simulink library "NSA_DEVS_LOGISTICS"  (R2025a)
settings: Solver=VariableStepAuto  StartTime=0.0  StopTime=10.0  RelTol=1e-3
libraries: $bdroot x9, NSA_DEVS_MATH_OPERATIONS x3, NSA_DEVS_ROUTING x1
settings Model: Creator=david  LastModifiedBy=peter
settings OptimizationCC: ReuseModelBlockBuffer=off
settings RTWCC: GPUComputeCapability=3.5

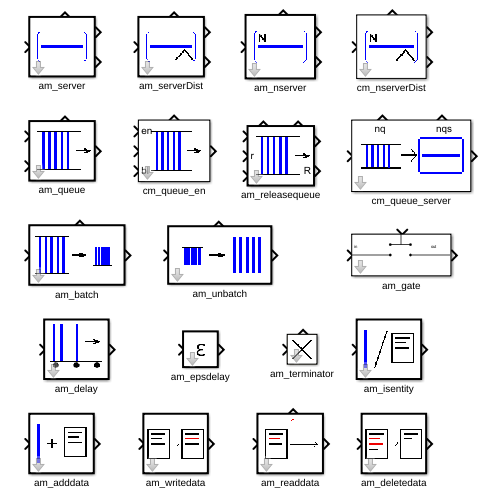
[thumbnail: Simulink's stored preview of the top-level diagram]
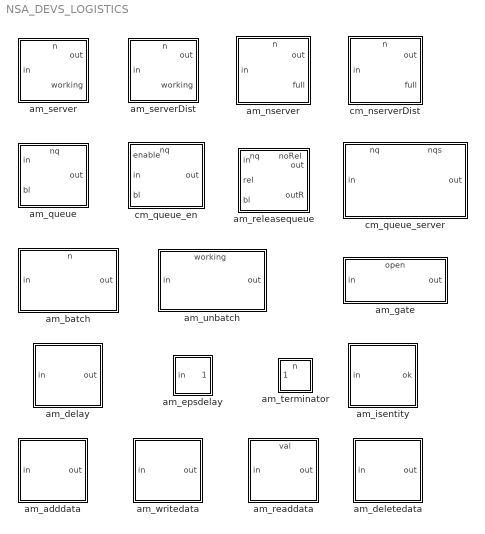
== system NSA_DEVS_LOGISTICS ==
  am_adddata : Subsystem  TreatAsAtomicUnit=on  mask(Adddata){fields=["name", "age"], values=["Peter", 42], numeric=[false, true], infield="id", tau=[0,1], debug=0}
      mask prompts: fields "field names"; values "field values"; numeric "flags to denote numeric values"; infield "field name of input value"
      mask help: Adds data fields to the input object.
      mask Help:
      | <p>Adds data fields to the input object.<br>
      | If the input is a struct, the new fields are added to the struct.
      | Otherwise a new struct is created and the incoming value is stored in an extra field.</p>
      | 
      | <p>Ports
      | <ul>
      | <li>inputs:
      |   <ul>
      |     <li>in: incoming value</li>
      |   </ul>
      | </li>
      | <li>outputs:
      |   <ul>
      |     <li>out: outgoing entity</li>
      |   </ul>
      | </li>
      | </ul>
      | </p>
      | 
      | <p>System Parameters
      | <ul>
      | <li>fields:  vector of new field names</li>
      | <li>values:  vector of corresponding values</li>
      | <li>numeric:  vector of booleans denoting numerical fields</li>
      | <li>infield:  field name for incoming value (if not a struct)</li>
      | <li>tau:   infinitesimal delay</li>
      | <li>debug: flag to enable debug information</li>
      | </ul>
      | </p>
      | 
      | <p>States
      | <ul>
      | <li>s:   running</li>
      | </ul>
      | </p>
      mask DialogControl Container4 Prompt: General
      mask DialogControl Container5 Prompt: Advanced
      mask Display: image('icon_adddata.png');
  am_batch : Subsystem  TreatAsAtomicUnit=on  mask(Batch){N=10, tau=[0,1], debug=0}
      mask prompts: N "batch size"
      mask help: Combine N entities to one batch entity.
      settings: PortSchema="{\"entries\":[{\"content\":{\"sides\":[{\"content\":{\"connectorIds\":[\"In1\"]},\"type\":\"ConnectorPlacement.EquallySpacedRectSide\",\"uuid\":\"8e15954b-329c-42af-8049-37e3c5654def\"},{\"content\":{\"connectorIds\":[\"Out1\"],\"side\":\"RIGHT\"},\"type\":\"ConnectorPlacement.EquallySpacedRectSide\",\"uuid\":\"63417118-70ef-43c0-aba5-016625c71a51\"},{\"content\":{\"connectorIds\":[\"Out2\"],\"side\":\"TOP\"},\"type\":\"ConnectorPlacement.EquallySpacedRectSide\",\"uuid\":\"b4e4d2cb-0431-4da8-a13e-061eb074f0ba\"}]},\"type\":\"ConnectorPlacement.EquallySpacedConnector\",\"uuid\":\"10cbbf1b-ecfb-492d-a1e3-9fcc3fe586bb\"}],\"packageUris\":[\"http://schema.mathworks.com/mf0/Connector/R2020b\"],\"version\":\"1.0\"}"
      mask Help:
      | <p>Combine N entities to one batch entity.</p>
      | 
      | <p>Ports
      | <ul>
      | <li>inputs:
      |   <ul>
      |     <li>in: incoming entities</li>
      |   </ul>
      | </li>
      | <li>outputs:
      |   <ul>
      |     <li>out: outgoing entities</li>
      |     <li>n: current internal batch size</li>
      |   </ul>
      | </li>
      | </ul>
      | </p>
      | 
      | <p>System Parameters
      | <ul>
      | <li>N:  number of input entities to be combined to one output batch</li>
      | <li>tau:   infinitesimal delay</li>
      | <li>debug: flag to enable debug information</li>
      | </ul>
      | </p>
      | 
      | <p>States
      | <ul>
      | <li>s:   running</li>
      | <li>E:  collection of incoming entities</li>
      | <li>n:  current number of internal entities</li>
      | </ul>
      | </p>
      mask DialogControl Container3 Prompt: General
      mask DialogControl Container4 Prompt: Advanced
      mask Display: image('icon_batch.png');
  am_delay : Subsystem  TreatAsAtomicUnit=on  mask(Delay){dt=[1,0], tau=[0,1], debug=0}
      mask prompts: dt "delay time"
      mask help: Delays the input signal by a constant amount.
      mask Help:
      | <p>Delays the input entities by a constant amount.</p>
      | 
      | <p>Ports
      | <ul>
      | <li>inputs:
      |   <ul>
      |     <li>in: incoming entities</li>
      |   </ul>
      | </li>
      | <li>outputs:
      |   <ul>
      |     <li>out: outgoing entities</li>
      |   </ul>
      | </li>
      | </ul>
      | </p>
      | 
      | <p>System Parameters
      | <ul>
      | <li>dt:  delay time</li>
      | <li>tau:   infinitesimal delay</li>
      | <li>debug: flag to enable debug information</li>
      | </ul>
      | </p>
      | 
      | <p>States
      | <ul>
      | <li>s:   running</li>
      | <li>E:  waiting input values, <br>E(i).x = value, E(i).e = remaining waiting time</li>
      | </ul>
      | </p>
      mask DialogControl Container4 Prompt: General
      mask DialogControl Container5 Prompt: Advanced
      mask Display: image('icon_delay.png');
  am_deletedata : Subsystem  TreatAsAtomicUnit=on  mask(Deletedata){fields="tS", tau=[0,1], debug=0}
      mask prompts: fields "fields to delete"
      mask help: Deletes data fields from the input object.
      mask Help:
      | <p>Deletes data fields from the input object.</p>
      | 
      | <p>Ports
      | <ul>
      | <li>inputs:
      |   <ul>
      |     <li>in: incoming entity</li>
      |   </ul>
      | </li>
      | <li>outputs:
      |   <ul>
      |     <li>out: outgoing entity</li>
      |   </ul>
      | </li>
      | </ul>
      | </p>
      | 
      | <p>System Parameters
      | <ul>
      | <li>fields:   vector of field names to be deleted</li>
      | <li>tau:   infinitesimal delay</li>
      | <li>debug: flag to enable debug information</li>
      | </ul>
      | </p>
      | 
      | <p>States
      | <ul>
      | <li>s:   running</li>
      | </ul>
      | </p>
      mask DialogControl Container4 Prompt: General
      mask DialogControl Container5 Prompt: Advanced
      mask Display: image('icon_deletedata.png');
  am_epsdelay : Subsystem  TreatAsAtomicUnit=on  mask(EpsDelay){tau=[0,1], debug=0}
      mask help: Delays its input by an infinitesimal amount.
      mask Help:
      | <p>Delays its input by an infinitesimal amount.</p>
      | 
      | <p>Ports
      | <ul>
      | <li>inputs:
      |   <ul>
      |     <li>in: incoming value or entity</li>
      |   </ul>
      | </li>
      | <li>outputs:
      |   <ul>
      |     <li>out: outgoing value or entity</li>
      |   </ul>
      | </li>
      | </ul>
      | </p>
      | 
      | <p>System Parameters
      | <ul>
      | <li>debug: flag to enable debug information</li>
      | <li>tau:   infinitesimal delay</li>
      | </ul>
      | </p>
      | 
      | <p>States
      | <ul>
      | <li>s:   running</li>
      | </ul>
      | </p>
      mask DialogControl Container5 Prompt: Advanced
      mask Display: image('icon_epsdelay.png');
  am_gate : Subsystem  mask(Gate){isOpen0=false, tau_copy_copy=[0,1], debug_copy_copy=0}
      mask prompts: isOpen0 "initial value of isOpen"; tau_copy_copy "tau"; debug_copy_copy "debug"
      mask help: Sends input entities to output, if gate is open, otherwise entities "disappear".
      settings: PortSchema="{\"entries\":[{\"content\":{\"sides\":[{\"content\":{\"connectorIds\":[\"In1\"]},\"type\":\"ConnectorPlacement.EquallySpacedRectSide\",\"uuid\":\"9e91849d-6784-4c2c-85c5-1ae2d6674bd6\"},{\"content\":{\"connectorIds\":[\"Out1\"],\"side\":\"RIGHT\"},\"type\":\"ConnectorPlacement.EquallySpacedRectSide\",\"uuid\":\"66074a09-403a-4c81-afe9-07f004dde84b\"},{\"content\":{\"connectorIds\":[\"In2\"],\"side\":\"TOP\"},\"type\":\"ConnectorPlacement.EquallySpacedRectSide\",\"uuid\":\"075d8e34-2efa-4755-8a48-3c73e13f58a7\"}]},\"type\":\"ConnectorPlacement.EquallySpacedConnector\",\"uuid\":\"f5de08e4-7e6c-4daa-a2bd-e0535eca4f4f\"}],\"packageUris\":[\"http://schema.mathworks.com/mf0/Connector/R2020b\"],\"version\":\"1.0\"}"
      mask Help:
      | <p>Sends input entities to output, if gate is open, otherwise entities "disappear".</p>
      | 
      | <p>Ports
      | <ul>
      | <li>inputs:
      |   <ul>
      |     <li>in: incoming entities</li>
      |     <li>open: state of gate</li>
      |   </ul>
      | </li>
      | <li>outputs:
      |   <ul>
      |     <li>out: outgoing entities</li>
      |   </ul>
      | </li>
      | </ul>
      | </p>
      | 
      | <p>System Parameters
      | <ul>
      | <li>isOpen0: initial value of isOpen </li>
      | <li>debug: flag to enable debug information</li>
      | <li>tau:   infinitesimal delay</li>
      | </ul>
      | </p>
      | 
      | <p>States
      | <ul>
      | <li>isOpen:    basic state of gate (true = open, false = closed)</li>
      | </ul>
      | </p>
      mask DialogControl Container5 Prompt: General
      mask DialogControl Container6 Prompt: Advanced
  am_isentity : Subsystem  TreatAsAtomicUnit=on  mask(Isentity){tau=[0,1], debug=0}
      mask help: Checks, whether the incoming event describes an entity.
      mask Help:
      | <p>Checks, whether the incoming event describes an entity.</p>
      | 
      | <p>Ports
      | <ul>
      | <li>inputs:
      |   <ul>
      |     <li>in: incoming value</li>
      |   </ul>
      | </li>
      | <li>outputs:
      |   <ul>
      |     <li>ok: true, if incoming event describes an entity</li>
      |   </ul>
      | </li>
      | </ul>
      | </p>
      | 
      | <p>System Parameters
      | <ul>
      | <li>debug: flag to enable debug information</li>
      | <li>tau:   infinitesimal delay</li>
      | </ul>
      | </p>
      | 
      | <p>States
      | <ul>
      | <li>s:   running</li>
      | </ul>
      | </p>
      mask DialogControl Container5 Prompt: Advanced
      mask Display: image('icon_isentity.png');
  am_nserver : Subsystem  TreatAsAtomicUnit=on  mask(Server){N=2, tS=1.0, tsField="", tD=[0,2], tau=[0,1], debug=0}
      mask prompts: N "capacity"; tS "service time"; tsField "input field containing tS"
      mask help: Processes up to N entities, each with a service time tS.
      settings: PortSchema="{\"entries\":[{\"content\":{\"sides\":[{\"content\":{\"connectorIds\":[\"In1\"]},\"type\":\"ConnectorPlacement.EquallySpacedRectSide\",\"uuid\":\"5b183f90-fa7c-445f-8fcc-24f596b19ad3\"},{\"content\":{\"connectorIds\":[\"Out1\",\"Out2\"],\"side\":\"RIGHT\"},\"type\":\"ConnectorPlacement.EquallySpacedRectSide\",\"uuid\":\"38178c13-d678-4577-a6b9-5280f6db2632\"},{\"content\":{\"connectorIds\":[\"Out3\"],\"side\":\"TOP\"},\"type\":\"ConnectorPlacement.EquallySpacedRectSide\",\"uuid\":\"c2d9ca5e-efc6-4807-b8ad-a826c28aecf1\"}]},\"type\":\"ConnectorPlacement.EquallySpacedConnector\",\"uuid\":\"5cc057fe-c578-4b16-bb74-4fc14b24d767\"}],\"packageUris\":[\"http://schema.mathworks.com/mf0/Connector/R2020b\"],\"version\":\"1.0\"}"
      mask Help:
      | <p>Processes up to N entities, each with a service time tS.<br>
      |  tS is given as parameter or via an input field.</p>
      | 
      | <p>Ports
      | <ul>
      | <li>inputs:
      |   <ul>
      |     <li>in: incoming entity</li>
      |   </ul>
      | </li>
      | <li>outputs:
      |   <ul>
      |     <li>out: outgoing entity</li>
      |     <li>working: server state (true/false)</li>
      |     <li>n: current number of entities in server</li>
      |   </ul>
      | </li>
      | </ul>
      | </p>
      | 
      | <p>System Parameters
      | <ul>
      | <li>N:  capacity</li>
      | <li>tS:  service time</li>
      | <li>tsField: name of input field containing tS ("": use parameter)</li>
      | <li>debug: flag to enable debug information</li>
      | <li>tau:   infinitesimal delay</li>
      | </ul>
      | </p>
      | 
      | <p>States
      | <ul>
      | <li>s:   idle|working|emitting</li>
      | <li>E:  data of processed entities (Nx1)</li>
      | <li>sig:  exit times of processed entities (Nx2, since hyperreals)</li>
      | <li>qOut: list of outgoing entities</li>
      | </ul>
      | </p>
      mask DialogControl Container4 Prompt: General
      mask DialogControl Container5 Prompt: Advanced
      mask Display: image('icon_nserver.png');
  am_queue : Subsystem  TreatAsAtomicUnit=on  mask(Queue){tD=[0,2], tau=[0,1], debug=0}
      mask prompts: tD "delay time of the queuingFree state"
      mask help: FIFO queue with output of current queue length.
      settings: PortSchema="{\"entries\":[{\"content\":{\"sides\":[{\"content\":{\"connectorIds\":[\"In1\",\"In2\"]},\"type\":\"ConnectorPlacement.EquallySpacedRectSide\",\"uuid\":\"a540ed89-9b5d-441d-ada7-41a21a0b2235\"},{\"content\":{\"connectorIds\":[\"Out1\"],\"side\":\"RIGHT\"},\"type\":\"ConnectorPlacement.EquallySpacedRectSide\",\"uuid\":\"9c4633e5-6641-4191-bf3a-c71013e8ac94\"},{\"content\":{\"connectorIds\":[\"Out2\"],\"side\":\"TOP\"},\"type\":\"ConnectorPlacement.EquallySpacedRectSide\",\"uuid\":\"35d87cf5-8c85-4911-a506-7e26d958e780\"}]},\"type\":\"ConnectorPlacement.EquallySpacedConnector\",\"uuid\":\"f4845054-9a98-4389-a979-55340d26924f\"}],\"packageUris\":[\"http://schema.mathworks.com/mf0/Connector/R2020b\"],\"version\":\"1.0\"}"
      mask Help:
      | <p>FIFO queue with output of current queue length.</p>
      | 
      | <p>Ports
      | <ul>
      | <li>inputs:
      |   <ul>
      |     <li>in: incoming entities</li>
      |     <li>bl: new blocking status at output</li>
      |   </ul>
      | </li>
      | <li>outputs:
      |   <ul>
      |     <li>out: outgoing entities</li>
      |     <li>nq: queue length</li>
      |   </ul>
      | </li>
      | </ul>
      | </p>
      | 
      | <p>System Parameters
      | <ul>
      | <li>tD:  delay time of the queuingFree state</li>
      | <li>debug: flag to enable debug information</li>
      | <li>tau:   infinitesimal delay</li>
      | </ul>
      | </p>
      | 
      | <p>States
      | <ul>
      | <li>name:  object name</li>
      | <li>s:   emptyFree|emptyBlocked|queuingFree|queuingBlocked</li>
      | <li>q:  vector of queued entities</li>
      | </ul>
      | </p>
      mask DialogControl Container5 Prompt: Advanced
      mask Display: image('icon_queue.png');
  am_readdata : Subsystem  TreatAsAtomicUnit=on  mask(Readdata){field="fieldname", tau=[0,1], debug=0}
      mask prompts: field "field to read"
      mask help: Outputs value of a data field from the input entity.
      settings: PortSchema="{\"entries\":[{\"content\":{\"sides\":[{\"content\":{\"connectorIds\":[\"In1\"]},\"type\":\"ConnectorPlacement.EquallySpacedRectSide\",\"uuid\":\"af4f6e7f-4af3-4de3-ab26-fba0b0c6ecc4\"},{\"content\":{\"connectorIds\":[\"Out1\"],\"side\":\"RIGHT\"},\"type\":\"ConnectorPlacement.EquallySpacedRectSide\",\"uuid\":\"ccdbf49e-e606-4b9c-9d6c-043b910468ef\"},{\"content\":{\"connectorIds\":[\"Out2\"],\"side\":\"TOP\"},\"type\":\"ConnectorPlacement.EquallySpacedRectSide\",\"uuid\":\"5949fb50-bad2-4ec4-8482-cd36555d236b\"},{\"content\":{\"side\":\"BOTTOM\"},\"type\":\"ConnectorPlacement.EquallySpacedRectSide\",\"uuid\":\"de5f47d7-31e8-457e-80ce-253364143e4a\"}]},\"type\":\"ConnectorPlacement.EquallySpacedConnector\",\"uuid\":\"b993aaba-7166-4556-9786-ee288ec6cbc2\"}],\"packageUris\":[\"http://schema.mathworks.com/mf0/Connector/R2020b\"],\"version\":\"1.0\"}"
      mask Help:
      | <p>Outputs value of a data field from the input entity.</p>
      | 
      | <p>Ports
      | <ul>
      | <li>inputs:
      |   <ul>
      |     <li>in: incoming entity</li>
      |   </ul>
      | </li>
      | <li>outputs:
      |   <ul>
      |     <li>out: outgoing entity</li>
      |     <li>val: value read from the input entity</li>
      |   </ul>
      | </li>
      | </ul>
      | </p>
      | 
      | <p>System Parameters
      | <ul>
      | <li>field:   field name to be read</li>
      | <li>tau:   infinitesimal delay</li>
      | <li>debug: flag to enable debug information</li>
      | </ul>
      | </p>
      | 
      | <p>States
      | <ul>
      | <li>s:   running</li>
      | </ul>
      | </p>
      mask DialogControl Container3 Prompt: General
      mask DialogControl Container4 Prompt: Advanced
      mask Display: image('icon_readdata.png');
  am_releasequeue : Subsystem  TreatAsAtomicUnit=on  mask(ReleaseQueue){useSingleElementBatch=false, tD=[0,2], tau=[0,1], debug=0}
      mask prompts: useSingleElementBatch "use batch for single released element"; tD "delay time of the queuingFree state"
      mask help:
      | FIFO queue with output of current queue length.
      | Outputs selected entities through output outR, when a release control signal arrives at input rel.
      settings: PortSchema="{\"entries\":[{\"content\":{\"sides\":[{\"content\":{\"connectorIds\":[\"In1\",\"In2\",\"In3\"]},\"type\":\"ConnectorPlacement.EquallySpacedRectSide\",\"uuid\":\"13ed37bb-b7d7-4a3e-85e9-ca5352af307b\"},{\"content\":{\"connectorIds\":[\"Out1\",\"Out2\"],\"side\":\"RIGHT\"},\"type\":\"ConnectorPlacement.EquallySpacedRectSide\",\"uuid\":\"9ca67023-fccb-4996-bf1d-9867d6e863f3\"},{\"content\":{\"connectorIds\":[\"Out3\",\"Out4\"],\"side\":\"TOP\"},\"type\":\"ConnectorPlacement.EquallySpacedRectSide\",\"uuid\":\"17642d09-3124-48e9-8501-bdbb934ba296\"}]},\"type\":\"ConnectorPlacement.EquallySpacedConnector\",\"uuid\":\"cd467e12-51be-446a-93c9-f234b6f2971a\"}],\"packageUris\":[\"http://schema.mathworks.com/mf0/Connector/R2020b\"],\"version\":\"1.0\"}"
      mask Help:
      | <p>FIFO queue with output of current queue length.<br>
      |   Outputs selected entities through output outR, when a release control entity arrives at input rel.<br>
      |   Type of the control entity:
      |   <ul>
      |   <li>rel = {name, value} → entities with attribute name=value are released<br>
      |   <li>special name "queuePosition_" → releases entities at given queue position<br>
      |   <li>value > 0 → counts from front end, value < 0 → counts from back end</p>
      |   </ul>
      | 
      | <p>Ports
      | <ul>
      | <li>inputs:
      |   <ul>
      |     <li>in: incoming entities</li>
      |     <li>bl: new blocking status at output</li>
      |     <li>rel: release control input</li>
      |   </ul>
      | </li>
      | <li>outputs:
      |   <ul>
      |     <li>out: outgoing entities</li>
      |     <li>outR: released entities as batch. Single entity is output directly, except when useSingleElementBatch = true</li>
      |     <li>nq: queue length</li>
      |     <li>noRel: true, if no entities are released at rel input</li>
      |   </ul>
      | </li>
      | </ul>
      | </p>
      | 
      | <p>System Parameters
      | <ul>
      | <li>name:  object name</li>
      | <li>useSingleElementBatch: flag with default = false, set it to true, when expecting one or more entities at outR</li>
      | <li>tD:  delay time of the queuingFree state</li>
      | <li>tau:   infinitesimal delay</li>
      | <li>debug: flag to enable debug information</li>
      | </ul>
      | </p>
      | 
      | <p>States
      | <ul>
      | <li>phase:   Queuing|Releasing</li>
      | <li>phaseQ:   emptyFree|emptyBlocked|queuingFree|queuingBlocked</li>
      | <li>q:  vector of queued entities</li>
      | <li>qR:  vector of entities to release</li>
      | </ul>
      | </p>
      mask DialogControl Container4 Prompt: General
      mask DialogControl Container3 Prompt: Advanced
      mask Display:
      | image('icon_queue.png');
      | port_label('input', 2, 'r');
      | port_label('output', 2, 'R');
  am_server : Subsystem  TreatAsAtomicUnit=on  mask(Server){tS=1.0, tsField="", tau=[0,1], debug=0}
      mask prompts: tS "service time"; tsField "input field for tS"
      mask help:
      | Processes one entity in time tS.
      | tS is given as parameter or via an input field.
      settings: PortSchema="{\"entries\":[{\"content\":{\"sides\":[{\"content\":{\"connectorIds\":[\"In1\"]},\"type\":\"ConnectorPlacement.EquallySpacedRectSide\",\"uuid\":\"5b183f90-fa7c-445f-8fcc-24f596b19ad3\"},{\"content\":{\"connectorIds\":[\"Out1\",\"Out2\"],\"side\":\"RIGHT\"},\"type\":\"ConnectorPlacement.EquallySpacedRectSide\",\"uuid\":\"38178c13-d678-4577-a6b9-5280f6db2632\"},{\"content\":{\"connectorIds\":[\"Out3\"],\"side\":\"TOP\"},\"type\":\"ConnectorPlacement.EquallySpacedRectSide\",\"uuid\":\"c2d9ca5e-efc6-4807-b8ad-a826c28aecf1\"}]},\"type\":\"ConnectorPlacement.EquallySpacedConnector\",\"uuid\":\"5cc057fe-c578-4b16-bb74-4fc14b24d767\"}],\"packageUris\":[\"http://schema.mathworks.com/mf0/Connector/R2020b\"],\"version\":\"1.0\"}"
      mask Help:
      | <p>Processes one entity in time tS.<br>
      |    tS is given as parameter or via an input field.</p>
      | 
      | <p>Ports
      | <ul>
      | <li>inputs:
      |   <ul>
      |     <li>in: incoming entities</li>
      |   </ul>
      | </li>
      | <li>outputs:
      |   <ul>
      |     <li>out: outgoing entities</li>
      |     <li>working: server state (true/false)</li>
      |     <li>n: current number of entities in server</li>
      |   </ul>
      | </li>
      | </ul>
      | </p>
      | 
      | <p>System Parameters
      | <ul>
      | <li>tS:  service time</li>
      | <li>tsField: name of input field containing tS ("": use parameter)</li>
      | <li>debug: flag to enable debug information</li>
      | <li>tau:   infinitesimal delay</li>
      | </ul>
      | </p>
      | 
      | <p>States
      | <ul>
      | <li>s:   idle|busy</li>
      | <li>E:  id of processed entity</li>
      | <li>sig:  next switching time</li>
      | </ul>
      | </p>
      mask DialogControl Container4 Prompt: General
      mask DialogControl Container5 Prompt: Advanced
      mask Display: image('icon_server.png');
  am_serverDist : Subsystem  TreatAsAtomicUnit=on  mask(ServerDist){distName="Constant", distPara=[1], tau=[0,1], debug=0}
      mask prompts: distName "distribution name"; distPara "distribution parameters"
      mask help: Processes one entity in time tS, where tS is a random number with given distribution.
      settings: PortSchema="{\"entries\":[{\"content\":{\"sides\":[{\"content\":{\"connectorIds\":[\"In1\"]},\"type\":\"ConnectorPlacement.EquallySpacedRectSide\",\"uuid\":\"5b183f90-fa7c-445f-8fcc-24f596b19ad3\"},{\"content\":{\"connectorIds\":[\"Out1\",\"Out2\"],\"side\":\"RIGHT\"},\"type\":\"ConnectorPlacement.EquallySpacedRectSide\",\"uuid\":\"38178c13-d678-4577-a6b9-5280f6db2632\"},{\"content\":{\"connectorIds\":[\"Out3\"],\"side\":\"TOP\"},\"type\":\"ConnectorPlacement.EquallySpacedRectSide\",\"uuid\":\"c2d9ca5e-efc6-4807-b8ad-a826c28aecf1\"}]},\"type\":\"ConnectorPlacement.EquallySpacedConnector\",\"uuid\":\"5cc057fe-c578-4b16-bb74-4fc14b24d767\"}],\"packageUris\":[\"http://schema.mathworks.com/mf0/Connector/R2020b\"],\"version\":\"1.0\"}"
      mask Help:
      | <p>Processes one entity in time tS, where tS is a random number with given distribution.</p>
      | 
      | <p>Ports
      | <ul>
      | <li>inputs:
      |   <ul>
      |     <li>in: incoming entities</li>
      |   </ul>
      | </li>
      | <li>outputs:
      |   <ul>
      |     <li>out: outgoing entities</li>
      |     <li>working: server state (true/false)</li>
      |     <li>n: current number of entities in server</li>
      |   </ul>
      | </li>
      | </ul>
      | </p>
      | 
      | <p>Parameters
      | <ul>
      | <li>distName: distribution name (Constant/Exponential/Triangular)</li>
      | <li>distPara: vector with distribution parameters</li>
      |   <ul>
      |     <li>Constant: [value]</li>
      |     <li>Exponential: [mean value]</li>
      |     <li>Triangular: [minValue, mostValue, maxValue]</li>
      |   </ul>
      | <li>tau:   infinitesimal delay</li>
      | <li>debug: flag to enable debug information</li>
      | </ul>
      | </p>
      | 
      | <p>States
      | <ul>
      | <li>s:   idle|busy</li>
      | <li>E:  id of processed entity</li>
      | <li>tSNext: next service time</li>
      | <li>sig:  next switching time</li>
      | </ul>
      | </p>
      mask TypeOptions distName: "Constant" | "Exponential" | "Triangular"
      mask DialogControl Container4 Prompt: General
      mask DialogControl distPara Tooltip: vector with dist specific  paras
      mask DialogControl Container5 Prompt: Advanced
      mask Display: image('icon_serverDist.png');
  am_terminator : Subsystem  mask(Terminator){tau=[0,1], debug=0}
      mask help:
      | Terminates incoming entities.
      | Outputs total number of incoming entities.
      settings: PortSchema="{\"entries\":[{\"content\":{\"sides\":[{\"content\":{\"connectorIds\":[\"In1\"]},\"type\":\"ConnectorPlacement.EquallySpacedRectSide\",\"uuid\":\"49bb8e9f-90f2-4275-9611-e25e817b13b5\"},{\"content\":{\"side\":\"RIGHT\"},\"type\":\"ConnectorPlacement.EquallySpacedRectSide\",\"uuid\":\"c18d105c-f57d-4a33-ac03-be83593b975c\"},{\"content\":{\"connectorIds\":[\"Out1\"],\"side\":\"TOP\"},\"type\":\"ConnectorPlacement.EquallySpacedRectSide\",\"uuid\":\"7eb98b6c-4be6-42dc-bb19-f921c03197ce\"}]},\"type\":\"ConnectorPlacement.EquallySpacedConnector\",\"uuid\":\"cb24cab6-e2b4-4253-bbca-dbf3db4c22b3\"}],\"packageUris\":[\"http://schema.mathworks.com/mf0/Connector/R2020b\"],\"version\":\"1.0\"}"
      mask Help:
      | <p>Terminates incoming entities.<br>
      | Outputs total number of incoming entities..</p>
      | 
      | <p>Ports
      | <ul>
      | <li>inputs:
      |   <ul>
      |     <li>in: incoming value</li>
      |   </ul>
      | </li>
      | <li>outputs:
      |   <ul>
      |     <li>n: total number of arrived entities</li>
      |   </ul>
      | </li>
      | </ul>
      | </p>
      | 
      | <p>System Parameters
      |  <ul>
      | <li>name:  object name</li>
      | <li>debug: flag to enable debug information</li>
      | <li>tau:   infinitesimal delay</li>
      | </ul>
      | </p>
      | 
      |  <p>States
      | <ul>
      | <li>name:  object name</li>
      | <li>s:   running</li>
      | <li>n:   total number of arrived entities</li>
      | <li>E:  last incoming value</li>
      | </ul>
      | </p>
      mask DialogControl Container3 Prompt: Advanced
      mask Display: image('icon_terminator.png');
  am_unbatch : Subsystem  TreatAsAtomicUnit=on  mask(Unbatch){tD=[0,2], tau=[0,1], debug=0}
      mask prompts: tD "time delay between outgoing entities of a batch"
      mask help: Unbatches the incoming batch entity.
      settings: PortSchema="{\"entries\":[{\"content\":{\"sides\":[{\"content\":{\"connectorIds\":[\"In1\"]},\"type\":\"ConnectorPlacement.EquallySpacedRectSide\",\"uuid\":\"699a685a-82e4-4da2-bfa9-e0858b917d6d\"},{\"content\":{\"connectorIds\":[\"Out1\"],\"side\":\"RIGHT\"},\"type\":\"ConnectorPlacement.EquallySpacedRectSide\",\"uuid\":\"5f2f7699-5233-4ca6-a241-8c900520435d\"},{\"content\":{\"connectorIds\":[\"Out2\"],\"side\":\"TOP\"},\"type\":\"ConnectorPlacement.EquallySpacedRectSide\",\"uuid\":\"48eec5c3-897c-4cbf-97be-4b70a690821b\"}]},\"type\":\"ConnectorPlacement.EquallySpacedConnector\",\"uuid\":\"07bc65d6-d200-436f-b4c9-be7513d1d0e2\"}],\"packageUris\":[\"http://schema.mathworks.com/mf0/Connector/R2020b\"],\"version\":\"1.0\"}"
      mask Help:
      | <p>Unbatches the incoming batch entity.</p>
      | 
      | <p>Ports
      | <ul>
      | <li>inputs:
      |   <ul>
      |     <li>in: incoming batch entity</li>
      |   </ul>
      | </li>
      | <li>outputs:
      |   <ul>
      |     <li>out: outgoing unbatched entities</li>
      |     <li>working: true if processing batch</li>
      |   </ul>
      | </li>
      | </ul>
      | </p>
      | 
      | <p>System Parameters
      | <ul>
      | <li>tD:  time delay between outgoing entities of a batch</li>
      | <li>tau:   infinitesimal delay</li>
      | <li>debug: flag to enable debug information</li>
      | </ul>
      | </p>
      | 
      | <p>States
      | <ul>
      | <li>s:   idle|busy</li>
      | <li>E:  incoming batch entity</li>
      | <li>n:   number of next outgoing entity</li>
      | </ul>
      | </p>
      mask DialogControl Container3 Prompt: Advanced
      mask Display: image('icon_unbatch.png');
  am_writedata : Subsystem  TreatAsAtomicUnit=on  mask(Writedata){inFields="inField", outField="outField", changeFunc="out = in(1) + rand();", tau=[0,1], debug=0}
      mask prompts: inFields "input field names"; outField "output field name"; changeFunc "changing function"
      mask help: Changes value of an incoming data field using values from other fields.
      mask Help:
      | <p>Changes value of an incoming data field using values from other fields.<br>
      | If an incoming entity has no corresponding field, it passes unchanged.</p>
      | 
      | <p>Ports
      | <ul>
      | <li>inputs:
      |   <ul>
      |     <li>in: incoming entity</li>
      |   </ul>
      | </li>
      | <li>outputs:
      |   <ul>
      |     <li>out: outgoing entity</li>
      |   </ul>
      | </li>
      | </ul>
      | </p>
      | 
      | <p>System Parameters
      | <ul>
      | <li>inFields:   field names that are used in change function</li>
      | <li>outField:   name of field, whose value is being changed</li>
      | <li>changeFunc: changing function of the form "val = f(v(i));"</li>
      | <li>tau:   infinitesimal delay</li>
      | <li>debug: flag to enable debug information</li>
      | </ul>
      | </p>
      | 
      | <p>States
      | <ul>
      | <li>s:   running</li>
      | </ul>
      | </p>
      mask DialogControl Container4 Prompt: General
      mask DialogControl Container5 Prompt: Advanced
      mask Display: image('icon_writedata.png');
  cm_nserverDist : Subsystem  mask(ExpNServer){N=3, distName="Exponential", distPara=[1], fieldname="tS", tD=[0,2], tau=[0,1], debug=0}
      mask prompts: N "capacity"; distName "distribution name"; distPara "distribution parameters"; fieldname "internal field name"
      mask help: N-server with randomly distributed service times, according to chosen distribution.
      settings: PortSchema="{\"entries\":[{\"content\":{\"sides\":[{\"content\":{\"connectorIds\":[\"In1\"]},\"type\":\"ConnectorPlacement.EquallySpacedRectSide\",\"uuid\":\"eca6e159-4e27-4729-aa7d-b464d6fdfe1f\"},{\"content\":{\"connectorIds\":[\"Out1\",\"Out2\"],\"side\":\"RIGHT\"},\"type\":\"ConnectorPlacement.EquallySpacedRectSide\",\"uuid\":\"154720cd-ea47-4284-be2d-6f7191e664f3\"},{\"content\":{\"connectorIds\":[\"Out3\"],\"side\":\"TOP\"},\"type\":\"ConnectorPlacement.EquallySpacedRectSide\",\"uuid\":\"b4b8fc0a-007a-4dc1-bdd8-8084dfb2c8c4\"}]},\"type\":\"ConnectorPlacement.EquallySpacedConnector\",\"uuid\":\"b2363db8-0b23-4f68-9440-40b4d3f16186\"}],\"packageUris\":[\"http://schema.mathworks.com/mf0/Connector/R2020b\"],\"version\":\"1.0\"}"
      mask TypeOptions distName: "Constant" | "Exponential" | "Triangular"
      mask DialogControl Container3 Prompt: General
      mask DialogControl distPara Tooltip: vector with dist specific  paras
      mask DialogControl Container4 Prompt: Advanced
      mask Display: image('icon_nserverDist.png');
  cm_queue_en : Subsystem  mask(QueueEn){tau=[0,1], debug=0}
      mask help: Queue with additionable enable input
      settings: PortSchema="{\"entries\":[{\"content\":{\"sides\":[{\"content\":{\"connectorIds\":[\"In1\",\"In2\",\"In3\"]},\"type\":\"ConnectorPlacement.EquallySpacedRectSide\",\"uuid\":\"049aff47-2d52-45a1-8cfe-c5a626c266e1\"},{\"content\":{\"connectorIds\":[\"Out1\"],\"side\":\"RIGHT\"},\"type\":\"ConnectorPlacement.EquallySpacedRectSide\",\"uuid\":\"d161dc95-73c9-457a-a499-61ffb49d079d\"},{\"content\":{\"connectorIds\":[\"Out2\"],\"side\":\"TOP\"},\"type\":\"ConnectorPlacement.EquallySpacedRectSide\",\"uuid\":\"1785de47-7f68-4a9a-b5e6-0a66b4c3b55d\"}]},\"type\":\"ConnectorPlacement.EquallySpacedConnector\",\"uuid\":\"6ecdd4d2-0921-4324-b437-891f6fdb2f7e\"}],\"packageUris\":[\"http://schema.mathworks.com/mf0/Connector/R2020b\"],\"version\":\"1.0\"}"
      mask Display:
      | image('icon_queue.png', [0.15,0,0,0,100,100]);
      | port_label('input', 1, 'en');
      | port_label('input', 3, 'bl');
  cm_queue_server : Subsystem  mask(QueueServer){ts=4.5, tau=[0,1], debug=0}
      mask help: Queue and server with outputs for entity numbers in queue and total
      settings: PortSchema="{\"entries\":[{\"content\":{\"sides\":[{\"content\":{\"connectorIds\":[\"In1\"]},\"type\":\"ConnectorPlacement.EquallySpacedRectSide\",\"uuid\":\"07fa0e51-8843-4ac9-8e94-884ae9a89d36\"},{\"content\":{\"connectorIds\":[\"Out1\"],\"side\":\"RIGHT\"},\"type\":\"ConnectorPlacement.EquallySpacedRectSide\",\"uuid\":\"0131ce69-7449-4362-9cfd-88c0df269334\"},{\"content\":{\"connectorIds\":[\"Out2\",\"Out3\"],\"side\":\"TOP\"},\"type\":\"ConnectorPlacement.EquallySpacedRectSide\",\"uuid\":\"407e2fdf-9916-4f3f-84c2-2a472bd1d59f\"}]},\"type\":\"ConnectorPlacement.EquallySpacedConnector\",\"uuid\":\"291a1c46-4425-425c-bba8-593c7bd17cc2\"}],\"packageUris\":[\"http://schema.mathworks.com/mf0/Connector/R2020b\"],\"version\":\"1.0\"}"
      mask DialogControl Container2 Prompt: General
      mask DialogControl Container3 Prompt: Advanced
      mask Display:
      | image('icon_queueserver.png');
      | text(0.20, 0.89, 'nq');
      | text(0.72, 0.89, 'nqs');

== system NSA_DEVS_LOGISTICS/am_adddata ==
  in : Inport
  out : Outport

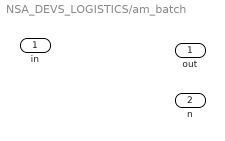
== system NSA_DEVS_LOGISTICS/am_batch ==
  in : Inport
  out : Outport
  n : Outport  Port=2

== system NSA_DEVS_LOGISTICS/am_delay ==
  in : Inport
  out : Outport

== system NSA_DEVS_LOGISTICS/am_deletedata ==
  in : Inport
  out : Outport

== system NSA_DEVS_LOGISTICS/am_epsdelay ==
  in : Inport
  out : Outport

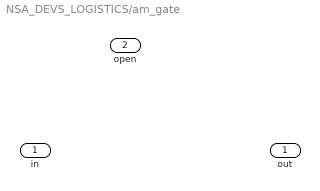
== system NSA_DEVS_LOGISTICS/am_gate ==
  in : Inport
  open : Inport  Port=2
  out : Outport

== system NSA_DEVS_LOGISTICS/am_isentity ==
  in : Inport
  ok : Outport

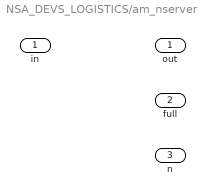
== system NSA_DEVS_LOGISTICS/am_nserver ==
  in : Inport
  out : Outport
  full : Outport  Port=2
  n : Outport  Port=3

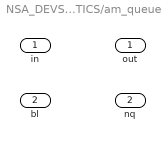
== system NSA_DEVS_LOGISTICS/am_queue ==
  in : Inport
  bl : Inport  Port=2
  out : Outport
  nq : Outport  Port=2

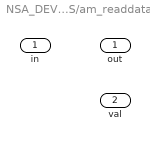
== system NSA_DEVS_LOGISTICS/am_readdata ==
  in : Inport
  out : Outport
  val : Outport  Port=2

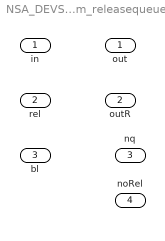
== system NSA_DEVS_LOGISTICS/am_releasequeue ==
  in : Inport
  rel : Inport  Port=2
  bl : Inport  Port=3
  out : Outport
  outR : Outport  Port=2
  nq : Outport  Port=3
  noRel : Outport  Port=4

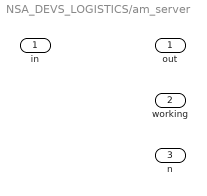
== system NSA_DEVS_LOGISTICS/am_server ==
  in : Inport
  out : Outport
  working : Outport  Port=2
  n : Outport  Port=3

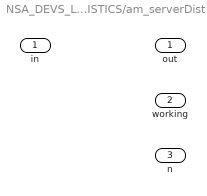
== system NSA_DEVS_LOGISTICS/am_serverDist ==
  in : Inport
  out : Outport
  working : Outport  Port=2
  n : Outport  Port=3

== system NSA_DEVS_LOGISTICS/am_terminator ==
  note: atomic = terminator(atomic_name, tau, debug);
  in : Inport
  n : Outport

== system NSA_DEVS_LOGISTICS/am_unbatch ==
  in : Inport
  out : Outport
  working : Outport  Port=2

== system NSA_DEVS_LOGISTICS/am_writedata ==
  in : Inport
  out : Outport

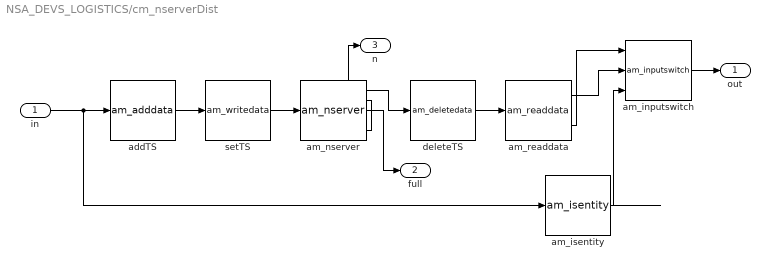
== system NSA_DEVS_LOGISTICS/cm_nserverDist ==
  in : Inport
  addTS : $bdroot/am_adddata  fields=fieldname  values="[\"1\"]"  numeric=[true]  infield="\"id\""  tau=0.1*tau  debug=debug
  am_inputswitch : NSA_DEVS_ROUTING/am_inputswitch  port0=1  tau=0.1*tau  debug=0
      settings: SourceProductName=Routing
  am_isentity : $bdroot/am_isentity  tau=0.1*tau  debug=0
  am_nserver : $bdroot/am_nserver  N=N  tS=1.0  tsField=fieldname  tD=tD  tau=0.5*tau  debug=debug
  am_readdata : $bdroot/am_readdata  field="\"id\""  tau=0.1*tau  debug=0
  deleteTS : $bdroot/am_deletedata  fields=fieldname  tau=0.1*tau  debug=debug
  setTS : $bdroot/am_writedata  inFields=[]  outField=fieldname  changeFunc="\"out = distributionFcn(\"\"\" + distName + \"\"\",  [\" + num2str(distPara) + \"]);\""  tau=0.1*tau  debug=debug
  out : Outport
  full : Outport  Port=2
  n : Outport  Port=3
  wires:
  addTS/1 -> setTS/1
  setTS/1 -> am_nserver/1
  am_nserver/1 -> deleteTS/1
  in/1 -> am_isentity/1, addTS/1
  am_nserver/3 -> n/1
  am_nserver/2 -> full/1
  deleteTS/1 -> am_readdata/1
  am_readdata/1 -> am_inputswitch/2
  am_readdata/2 -> am_inputswitch/1
  am_inputswitch/1 -> out/1
  am_isentity/1 -> am_inputswitch/3

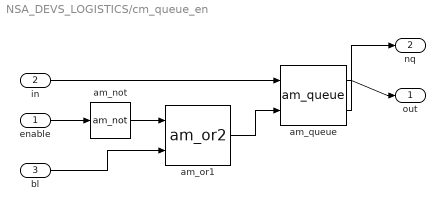
== system NSA_DEVS_LOGISTICS/cm_queue_en ==
  enable : Inport
  in : Inport  Port=2
  bl : Inport  Port=3
  am_not : NSA_DEVS_MATH_OPERATIONS/am_not  i0=true  tau_copy=[0,1]  debug_copy=0
      settings: SourceProductName=Math Operations
  am_or1 : NSA_DEVS_MATH_OPERATIONS/am_or2  i0=false  tau_copy=[0,1]  debug_copy=0
      settings: SourceProductName=Math Operations
  am_queue : $bdroot/am_queue  tD=tau+[0,1]  tau=tau  debug=debug
  out : Outport
  nq : Outport  Port=2
  wires:
  am_or1/1 -> am_queue/2
  am_not/1 -> am_or1/1
  bl/1 -> am_or1/2
  enable/1 -> am_not/1
  am_queue/2 -> nq/1
  am_queue/1 -> out/1
  in/1 -> am_queue/1

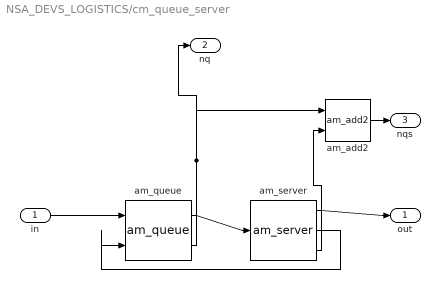
== system NSA_DEVS_LOGISTICS/cm_queue_server ==
  in : Inport
  am_add2 : NSA_DEVS_MATH_OPERATIONS/am_add2  tau=tau  debug=debug
      settings: SourceProductName=Math Operations
  am_queue : $bdroot/am_queue  tD=tau.*2  tau=tau  debug=debug
  am_server : $bdroot/am_server  tS=ts  tsField="\"\""  tau=tau  debug=debug
  out : Outport
  nq : Outport  Port=2
  nqs : Outport  Port=3
  wires:
  am_add2/1 -> nqs/1
  am_queue/2 -> nq/1, am_add2/1
  am_server/1 -> out/1
  am_server/2 -> am_queue/2
  in/1 -> am_queue/1
  am_queue/1 -> am_server/1
  am_server/3 -> am_add2/2
